simulink model "strRos2Matlab"  (R2022b)
settings: Solver=FixedStepAuto  StartTime=0.0  StopTime=inf  FixedStep=Ts  RelTol=1e-3
libraries: ros2lib x1
settings Model: Creator=System-10  LastModifiedBy=System-10

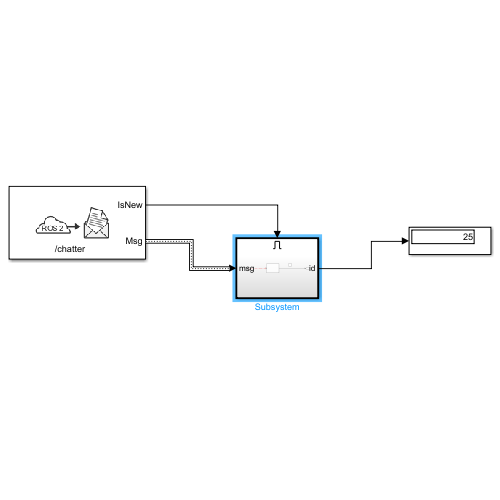
[thumbnail: Simulink's stored preview of the top-level diagram]
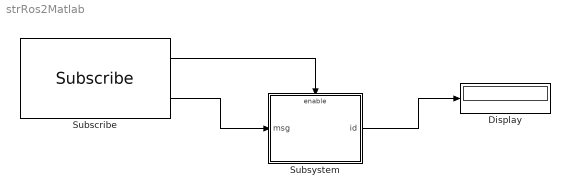
== system strRos2Matlab ==
  Display : Display
  Subscribe : ros2lib/Subscribe  topicSource=Specify your own  topic=/chatter  messageType=std_msgs/String  sampleTime=Ts  QOSHistory=Keep last  QOSDepth=1  QOSReliability=Reliable  QOSDurability=Volatile
      settings: LibrarySourceBlock=roslib/ROS 2/Subscribe
  Subsystem : Subsystem
  wires:
  Subscribe/2 -> Subsystem/1(msg)
  Subscribe/1 -> Subsystem/Enable
  Subsystem/1(id) -> Display/1

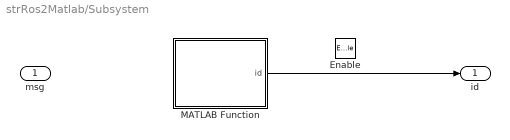
== system strRos2Matlab/Subsystem ==
  msg : Inport
  Enable : EnablePort
  MATLAB Function : MATLAB Function  TreatAsAtomicUnit=on
  id : Outport
  wires:
  MATLAB Function/1(id) -> id/1

== matlab function strRos2Matlab/Subsystem/MATLAB Function ==
  data: id output
function id = chatterCallback()
    
persistent data;
    if isempty(data)
        data = 0;
    end
    
    data = data+1;
    id = data;
end
